simulink model "Advanced_PID_final"  (R2023a)
settings: Solver=VariableStepAuto  StartTime=0.0  StopTime=86400  RelTol=1e-3
libraries: cstblocks x2, slpidlib x1
settings Model: Creator=Yuganshu Wadhwa  LastModifiedBy=Yuganshu Wadhwa

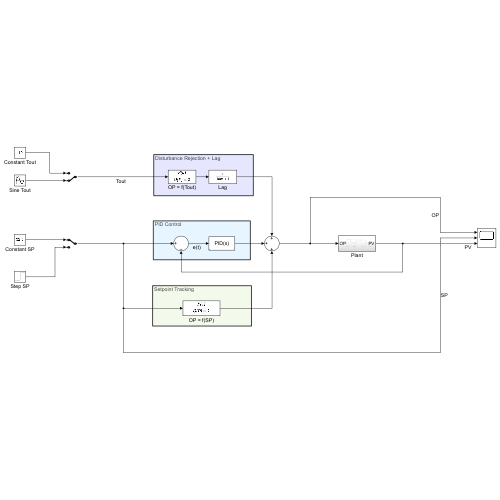
[thumbnail: Simulink's stored preview of the top-level diagram]
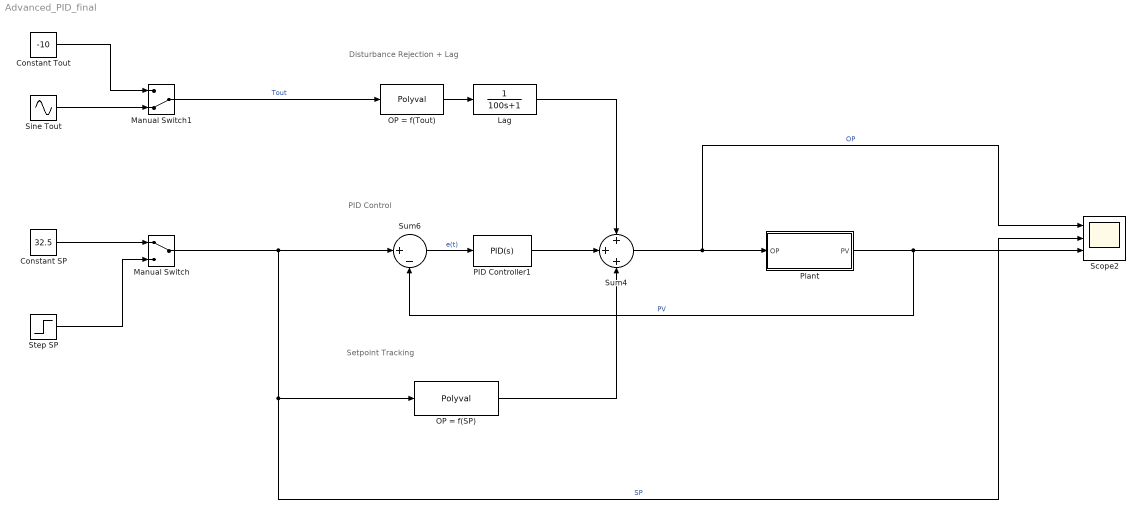
== system Advanced_PID_final ==
  note: Setpoint Tracking
  note: PID Control
  note: Disturbance Rejection + Lag
  Constant SP : Constant  Value=32.5
  Constant Tout : Constant  Value=-10
  Lag : TransferFcn  Denominator=[100 1]
  Manual Switch : ManualSwitch
  Manual Switch1 : ManualSwitch  CurrentSetting=0
  OP = f(SP) : Polyval  Coefs=[ +20.075, -1284.7, 20570]
  OP = f(Tout) : Polyval  Coefs=[ +0.5285, +0.2364, +16.302 ]
  PID Controller1 : slpidlib/PID Controller  Controller=PID  Form=Parallel  TimeDomain=Continuous-time  UseExternalTs=off  SampleTime=-1  IntegratorMethod=Forward Euler  FilterMethod=Forward Euler  ControllerParametersSource=internal  P=5  I=3  UseKiTs=off  D=0  N=1  UseFilter=on  TunerSelectOption=Transfer Function Based (PID Tuner App)  InitialConditionSource=internal  InitialConditionForIntegrator=0  InitialConditionForFilter=0  DifferentiatorICPrevScaledInput=0  ExternalReset=none  TrackingMode=off  Kt=1  LimitOutput=off  SatLimitsSource=internal  UpperSaturationLimit=100  LowerSaturationLimit=0  LinearizeAsGain=off  AntiWindupMode=back-calculation  Kb=1  LimitIntegrator=off  UpperIntegratorSaturationLimit=inf  LowerIntegratorSaturationLimit=-inf  POutMin=[]  POutMax=[]  IOutMin=[]  IOutMax=[]  DOutMin=[]  DOutMax=[]  NOutMin=[]  NOutMax=[]  SumOutMin=[]  SumOutMax=[]  SaturationOutMin=[]  SaturationOutMax=[]  PParamMin=[]  PParamMax=[]  IParamMin=[]  IParamMax=[]  DParamMin=[]  DParamMax=[]  NParamMin=[]  NParamMax=[]  KbParamMin=[]  KbParamMax=[]  KtParamMin=[]  KtParamMax=[]  KbOutMin=[]  KbOutMax=[]  KtOutMin=[]  KtOutMax=[]  IntegratorOutMin=[]  IntegratorOutMax=[]  FilterOutMin=[]  FilterOutMax=[]  SumI1OutMin=[]  SumI1OutMax=[]  SumI2OutMin=[]  SumI2OutMax=[]  SumI3OutMin=[]  SumI3OutMax=[]  SumI4OutMin=[]  SumI4OutMax=[]  SumDOutMin=[]  SumDOutMax=[]  DifferentiatorOutMin=[]  DifferentiatorOutMax=[]  FilterDiffOutCoefMin=[]  FilterDiffOutCoefMax=[]  ReciprocalOutMin=[]  ReciprocalOutMax=[]  SumDenOutMin=[]  SumDenOutMax=[]  SumNumOutMin=[]  SumNumOutMax=[]  DivideOutMin=[]  DivideOutMax=[]  UdiffTsProdOutMin=[]  UdiffTsProdOutMax=[]  NTsProdOutMin=[]  NTsProdOutMax=[]  UintegralTsProdOutMin=[]  UintegralTsProdOutMax=[]  UngainTsProdOutMin=[]  UngainTsProdOutMax=[]  ClampingZeroOutDataTypeStr=Inherit: Inherit via back propagation  ClampingZeroOutMin=[]  ClampingZeroOutMax=[]  FilterDenConstantOutDataTypeStr=Inherit: Inherit via back propagation  FilterDenConstantOutMin=[]  FilterDenConstantOutMax=[]  PCopyOutDataTypeStr=Inherit: Inherit via back propagation  PCopyOutMin=[]  PCopyOutMax=[]  NCopyOutDataTypeStr=Inherit: Inherit via back propagation  NCopyOutMin=[]  NCopyOutMax=[]  IntegratorContinuousStateAttributes=''  IntegratorStateMustResolveToSignalObject=off  IntegratorRTWStateStorageClass=Auto  FilterContinuousStateAttributes=''  FilterStateMustResolveToSignalObject=off  FilterRTWStateStorageClass=Auto  ParallelPVariant=InternalParameters  IdealPVariant=Disabled  IVariant=InternalParameters  DVariant=InternalParameters  IntegratorVariant=Continuous  SatVariant=Disabled  AWVariant=Passthrough  PCopyVariant=Disabled  TRVariant=Disabled  FdbkBlocksVariant=Forward  IdealPFdbkVariant=Disabled  SatFdbkVariant=Disabled  DerivativeFilterVariant=ContFilter  NVariant=InternalParameters  NCopyVariant=Disabled  FilterICVariant=InternalICsFilter  IntegratorICVariant=InternalICs  ExternalResetVariant=Disabled  TRSumVariant=Passthrough  SumFdbkVariant=Disabled  SumVariant=Sum_PID  TsampFilterVariant=InternalTs  TsampNgainVariant=Passthrough  TsampIntegralVariant=Disabled_SignalSpec  ExternalSaturationOutDataTypeStr=Inherit: Same as second input
  Plant : Subsystem
  Scope2 : Scope  NumInputPorts=3
  Sine Tout : Sin  Amplitude=6  Bias=-4  Frequency=(3.472e-05)*2*pi  SampleTime=0
  Step SP : Step  Time=500  Before=32  After=33.5  SampleTime=0
  Sum4 : Sum  Inputs=+++
  Sum6 : Sum  Inputs=|+-
  wires:
  OP = f(Tout)/1 -> Lag/1
  Sum4/1 -> Scope2/1, Plant/1(OP)  "OP"
  Step SP/1 -> Manual Switch/2
  Sine Tout/1 -> Manual Switch1/2
  Manual Switch/1 -> Sum6/1, OP = f(SP)/1, Scope2/2  "SP"
  Constant Tout/1 -> Manual Switch1/1
  Constant SP/1 -> Manual Switch/1
  Manual Switch1/1 -> OP = f(Tout)/1  "Tout"
  Sum6/1 -> PID Controller1/1  "e(t)"
  OP = f(SP)/1 -> Sum4/3
  Plant/1(PV) -> Scope2/3, Sum6/2  "PV"
  Lag/1 -> Sum4/1
  PID Controller1/1 -> Sum4/2

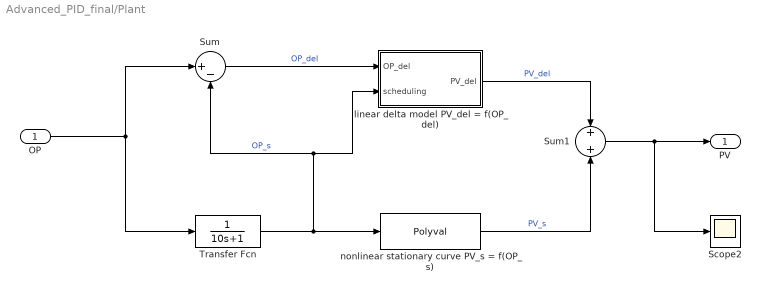
== system Advanced_PID_final/Plant ==
  OP : Inport
  Scope2 : Scope
  Sum : Sum  Inputs=|+-
  Sum1 : Sum  Inputs=+|+
  Transfer Fcn : TransferFcn  Denominator=[10 1]
  "linear delta model PV_del = f(OP_del) " : Subsystem
  nonlinear stationary curve PV_s = f(OP_s) : Polyval  Coefs=[ -0.0004, +0.0693, +30.896 ]
  PV : Outport
  wires:
  nonlinear stationary curve PV_s = f(OP_s)/1 -> Sum1/2  "PV_s"
  "linear delta model PV_del = f(OP_del) "/1(PV_del) -> Sum1/1  "PV_del"
  Sum1/1 -> Scope2/1, PV/1
  Sum/1 -> "linear delta model PV_del = f(OP_del) "/1(OP_del)  "OP_del"
  OP/1 -> Sum/1, Transfer Fcn/1
  Transfer Fcn/1 -> Sum/2, "linear delta model PV_del = f(OP_del) "/2(scheduling), nonlinear stationary curve PV_s = f(OP_s)/1  "OP_s"

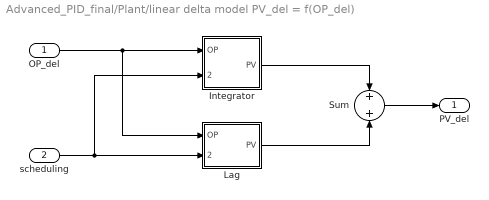
== system Advanced_PID_final/Plant/linear delta model PV_del = f(OP_del)  ==
  OP_del : Inport
  scheduling : Inport  Port=2
  Integrator : Subsystem
  Lag : Subsystem
  Sum : Sum  Inputs=+|+
  PV_del : Outport
  wires:
  Lag/1(PV) -> Sum/2
  Sum/1 -> PV_del/1
  scheduling/1 -> Integrator/2(scheduling), Lag/2(scheduling)
  OP_del/1 -> Lag/1(OP), Integrator/1(OP)
  Integrator/1(PV) -> Sum/1

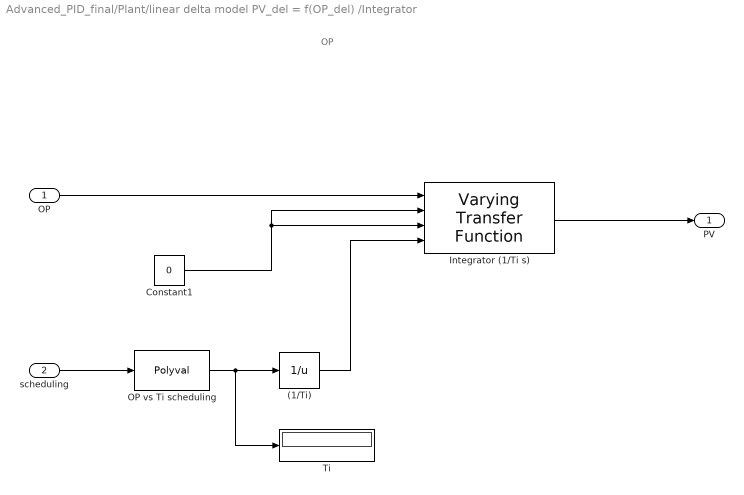
== system Advanced_PID_final/Plant/linear delta model PV_del = f(OP_del) /Integrator ==
  note: OP
  OP : Inport
  scheduling : Inport  Port=2
  (1/Ti) : Math  Operator=reciprocal
  Constant1 : Constant  Value=0
  Integrator (1/Ti s) : cstblocks/Linear Parameter Varying/Varying Transfer Function  N=1  Feedthrough=on
  OP vs Ti scheduling : Polyval  Coefs=[ +0.3812, -72.91, +4942.1, -110789, +1e+06 ]
  Ti : Display
  PV : Outport
  wires:
  OP/1 -> Integrator (1/Ti s)/1
  Constant1/1 -> Integrator (1/Ti s)/3, Integrator (1/Ti s)/2
  OP vs Ti scheduling/1 -> Ti/1, (1/Ti)/1
  Integrator (1/Ti s)/1 -> PV/1
  (1/Ti)/1 -> Integrator (1/Ti s)/4
  scheduling/1 -> OP vs Ti scheduling/1

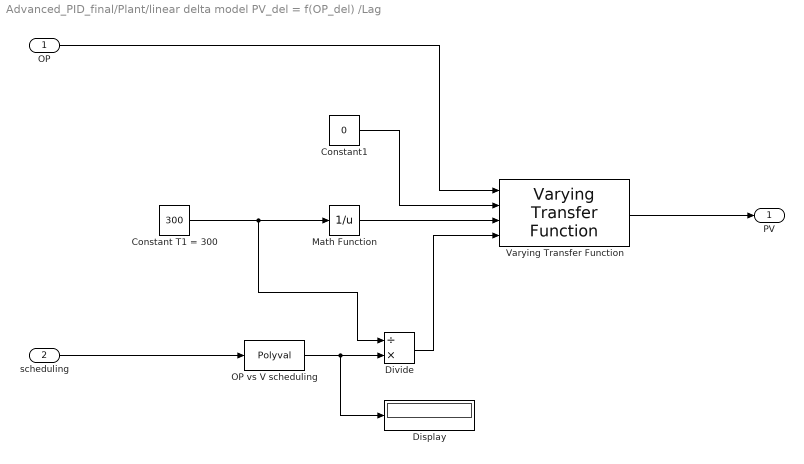
== system Advanced_PID_final/Plant/linear delta model PV_del = f(OP_del) /Lag ==
  OP : Inport
  scheduling : Inport  Port=2
  Constant T1 = 300 : Constant  Value=300
  Constant1 : Constant  Value=0
  Display : Display
  Divide : Product  Inputs=/*
  Math Function : Math  Operator=reciprocal
  OP vs V scheduling : Polyval  Coefs="[  -3e-7, +8e-5, -0.0065, 0.1944 ]"
  Varying Transfer Function : cstblocks/Linear Parameter Varying/Varying Transfer Function  N=1  Feedthrough=on
  PV : Outport
  wires:
  Divide/1 -> Varying Transfer Function/4
  Constant T1 = 300/1 -> Math Function/1, Divide/1
  Constant1/1 -> Varying Transfer Function/2
  OP/1 -> Varying Transfer Function/1
  OP vs V scheduling/1 -> Display/1, Divide/2
  Math Function/1 -> Varying Transfer Function/3
  Varying Transfer Function/1 -> PV/1
  scheduling/1 -> OP vs V scheduling/1
